simulink library "aerolibanim"  (R2015a)
settings: Solver=ode45  SolverMode=SingleTasking  StartTime=0.0  StopTime=10.0  RelTol=1e-3
PostLoadFcn:
  | load_system('aerolibv1')
  | setsysloc('aerolibv1')
undefined symbols (not defined in the file or in its folder): aeroicon
Description:
  | Aerospace Blockset Library: MATLAB-Based Animation
settings Model: FPTRunName=Active  ExtModeAutoUpdateStatusClock=off  Creator=The MathWorks Inc.  LastModifiedBy=Ali Muksin
settings DataIOCC: SignalLoggingSaveFormat=ModelDataLogs
settings OptimizationCC: BlockReduction=off  BooleanDataType=off  ExpressionDepthLimit=2147483647  EfficientMapNaN2IntZero=off
settings DebuggingCC: SaveWithParameterizedLinksMsg=none  UnderspecifiedInitializationDetection=Classic  MergeDetectMultiDrivingBlocksExec=none  SignalResolutionControl=TryResolveAllWithWarning  FcnCallInpInsideContextMsg=UseLocalSettings  StateNameClashWarn=warning  StrictBusMsg=Warning
settings HardwareCC: TargetUnknown=on
settings GRTTargetCC: CombineOutputUpdateFcns=off  GRTInterface=on

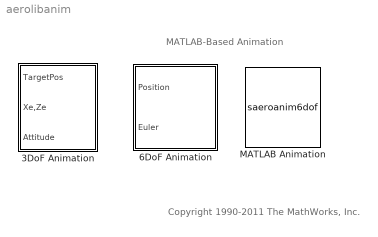
== system aerolibanim ==
  note: MATLAB-Based Animation
  note: Copyright 1990-2011 The MathWorks, Inc.
  3DoF Animation : Subsystem  TreatAsAtomicUnit=on  SimViewingDevice=on  mask(3DoF_Animation){u1=[0 5000 -2000 2000 -5050 -3050], u2=0.05, u3=1.0, u5=Fixed position, u6=[2000 500 -3150], u7=10, u8=on}
      mask prompts: u1 "Axes limits [xmin xmax ymin ymax zmin zmax]:"; u2 "Time interval between updates:"; u3 "Size of craft displayed:"; u5 "Enter view:"; u6 "Position of camera [xc yc zc]:"; u7 "View angle:"; u8 "Enable animation"
      mask help:
      | Create a 3-D animated view of a three-degrees-of-freedom craft and its target, where X and Z target position (TargetPos), X and Z craft position (Xe,Ze), and craft attitude are inputs.
      |
      | Display parameters are in the same units of length as the input parameters.
      mask init:
      | Config.axes = u1;
      | Config.update = u2;
      | Config.craft = u3;
      | Config.camera_view = u5;
      | Config.camera_pos = u6;
      | Config.view = u7;
      | Config.Animenable = u8;
      | Config.Model = bdroot(gcb);
      mask Help: eval('asbhelp(''threedof_animation'')');
      mask TypeOptions u5: Fixed position | Cockpit | Fly alongside
      mask Display:
      | port_label('input',1,'x_{t},z_{t}','texmode','on');
      | port_label('input',2,'x_e,z_e','texmode','on');
      | port_label('input',3,'\theta','texmode','on');
      | [xp yp] = aeroimage('anim',gcbh);
      | patch(xp,yp)
  6DoF Animation : Subsystem  TreatAsAtomicUnit=on  SimViewingDevice=on  mask(6DoF_Animation){u1=[0 4000 -2000 2000 -5000 -3000], u2=0.1, u3=1.0, u4=[4000 0 -5000], u5=Fixed position, u6=[2000 500 -3150], u7=10, u8=on}
      mask prompts: u1 "Axes limits [xmin xmax ymin ymax zmin zmax]:"; u2 "Time interval between updates:"; u3 "Size of craft displayed:"; u4 "Static object position [xp yp zp]:"; u5 "Enter view:"; u6 "Position of camera [xc yc zc]:"; u7 "View angle:"; u8 "Enable animation"
      mask help:
      | Create a 3-D animated view of a six-degrees-of-freedom craft, where X, Y, and Z craft position (Position) and craft Euler angles (Euler) are inputs.
      |
      | Display parameters are in the same units of length as the input parameters.
      mask init:
      | Config.axes = u1;
      | Config.update = u2;
      | Config.craft = u3;
      | Config.target = u4;
      | Config.camera_view = u5;
      | Config.camera_pos = u6;
      | Config.view = u7;
      | Config.Animenable = u8;
      | Config.Model = bdroot(gcb);
      mask Help: eval('asbhelp(''sixdof_animation'')');
      mask TypeOptions u5: Fixed position | Cockpit | Fly alongside
      mask Display:
      | port_label('input',1,'x_e','texmode','on');
      | port_label('input',2,'\phi \theta \psi','texmode','on');
      | [xp yp] = aeroimage('anim',gcbh);
      | patch(xp,yp)
  MATLAB Animation : S-Function  Tag=Matlab Animation 6 DOF  LoadFcn=aeroicon('aeroblkMatlabAnimation','load')  StartFcn=aeroicon('aeroblkMatlabAnimation','start')  FunctionName=saeroanim6dof  Parameters=Vehicles, SampleTime  mask(AeroMATLABAnimation){Vehicles=1, Geometries='astredwedge.mat', BoundingBoxCoordinates=[-50,50,-50,50,-50,50], CameraOffset=[-150,-50,0], CameraViewAngle=3, SampleTime=0.2, FigurePosition=[403,303,275,214], Open=off}
      mask prompts: Geometries "Geometries (use 'quotes' on filenames):"; BoundingBoxCoordinates "Bounding box coordinates:"; CameraOffset "Camera offset:"; CameraViewAngle "Camera view angle:"; SampleTime "Sample time:"; FigurePosition "Figure Position:"
      mask help:
      | Animate one or more vehicle geometries with XYZ position and euler angles through the specified bounding box,  camera offset, and field of view.  By default, the camera aim point is the position of the first body lagged dynamically to indicate motion.  The camera offset represents the distance from the camera aim point to the camera itself.  To update the camera parameters in the animation, first set the parameters then close and reopen the animation window.
      |
      | Vehicle geometries can be specified using a variable name, a cell array of variable names, a filename string with quotes 'mygeom.mat', or a mixed cell array of variable names and strings, e.g., {'file1.mat', 'file2.mat', 'file3.ac', geomVar }.  Currently, geometries specified in variables must exist in the MATLAB workspace and file names must exist in the current directory or be on the MATLAB path.
      mask init:
      | bh = gcbh;
      | [xp,yp] = aeroimage('anim',gcbh);
      | xp = xp+0.2;
      | yp = yp;
      | ud = get_param(bh,'UserData');
      | ud.CameraOffset = CameraOffset;
      | ud.BoundingBoxCoordinates = BoundingBoxCoordinates;
      | ud.CameraViewAngle = CameraViewAngle;
      | ud.Geometries = Geometries;
      | ud.BlockHandle = bh;
      | ud.Id = '6DOFcpp';
      | set_param(bh,'UserData',ud);
      | aeroicon('aeroblkMatlabAnimation','icon')
      settings: DeleteFcn=aeroicon('aeroblkMatlabAnimation','delete')  PreSaveFcn=aeroicon('aeroblkMatlabAnimation','presave')  NameChangeFcn=aeroicon('aeroblkMatlabAnimation','namechange')  DestroyFcn=aeroicon('aeroblkMatlabAnimation','delete')  OpenFcn=aeroicon('aeroblkMatlabAnimation','open')
      mask Help: eval('asbhelp(''matlab_animation'')');
      mask TypeOptions Vehicles: 1 | 2 | 3 | 4 | 5 | 6 | 7 | 8 | 9 | 10
      mask Display:
      | port_label('input',1,'1.X_e','texmode','on')
      | port_label('input',2,'1.\phi \theta \psi','texmode','on')
      | patch(xp,yp)

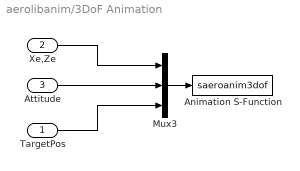
== system aerolibanim/3DoF Animation ==
  TargetPos : Inport
  Xe,Ze : Inport  Port=2
  Attitude : Inport  Port=3
  Animation S-Function : S-Function  FunctionName=saeroanim3dof  Parameters=Config
  Mux3 : Mux  Inputs=3
  wires:
  Mux3/1 -> Animation S-Function/1
  TargetPos/1 -> Mux3/3
  Attitude/1 -> Mux3/2
  Xe,Ze/1 -> Mux3/1

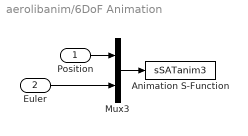
== system aerolibanim/6DoF Animation ==
  Position : Inport
  Euler : Inport  Port=2
  Animation S-Function : S-Function  FunctionName=sSATanim3  Parameters=Config
  Mux3 : Mux  Inputs=2
  wires:
  Euler/1 -> Mux3/2
  Position/1 -> Mux3/1
  Mux3/1 -> Animation S-Function/1
